simulink model "F_Transmission_loss"  (R2020a)
settings: Solver=VariableStepAuto  StartTime=0.0  StopTime=100000.0  RelTol=1e-3
libraries: simulink x1
settings Model: Creator=Abdullah Abdelaziz  LastModifiedBy=Abdullah Abdelaziz

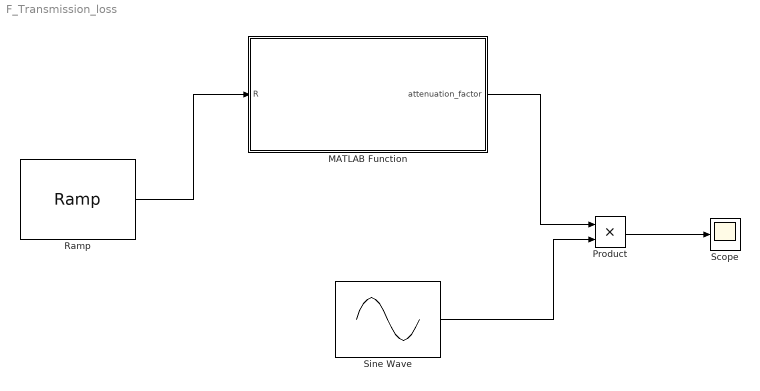
== system F_Transmission_loss ==
  MATLAB Function : MATLAB Function  TreatAsAtomicUnit=on
  Product : Product
  Ramp : simulink/Sources/Ramp  slope=50  start=5  InitialOutput=1
  Scope : Scope
  Sine Wave : Sin  Amplitude=50  SampleTime=0
  wires:
  Sine Wave/1 -> Product/2
  Product/1 -> Scope/1
  MATLAB Function/1(attenuation_factor) -> Product/1
  Ramp/1 -> MATLAB Function/1(R)

== matlab function F_Transmission_loss/MATLAB Function ==
  data: R input; attenuation_factor output
function attenuation_factor = calculate_attenuation(R)
% Calculates a linear attenuation factor based on transmission loss for a given range.
% This factor is suitable for multiplying with a signal to simulate loss.
%
% Input:
%   R = The range or distance in meters. Must be a positive number.
%
% Output:
%   attenuation_factor = A value between 0 and 1 representing the signal attenuation.

    % Error check: Ensure the range is a positive number.
    if R <= 0
        error('Range R must be a positive value.');
    end

    % 1. First, calculate the transmission loss in decibels (dB).
    loss_dB = 20 * log10(R);

    % 2. Convert the dB loss into a linear scaling factor for multiplication.
    attenuation_factor = 10^(-loss_dB / 20);
end
